simulink subsystem "GFDB"  (R2025b)
settings: Solver=VariableStepAuto  StartTime=0.0  StopTime=10.0  RelTol=1e-3
libraries: simulink x1
settings Model: Creator=diego  LastModifiedBy=ryanz
settings RTWCC: GPUComputeCapability=3.5

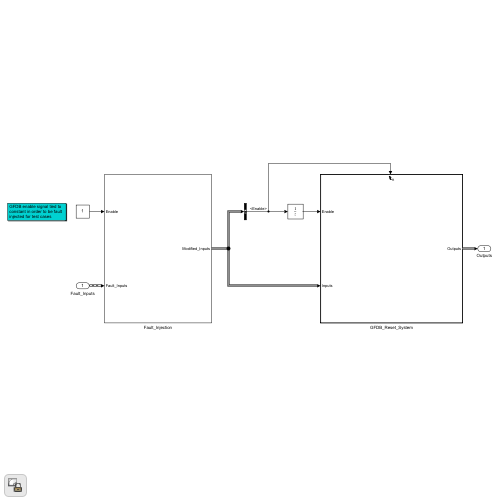
[thumbnail: Simulink's stored preview of the top-level diagram]
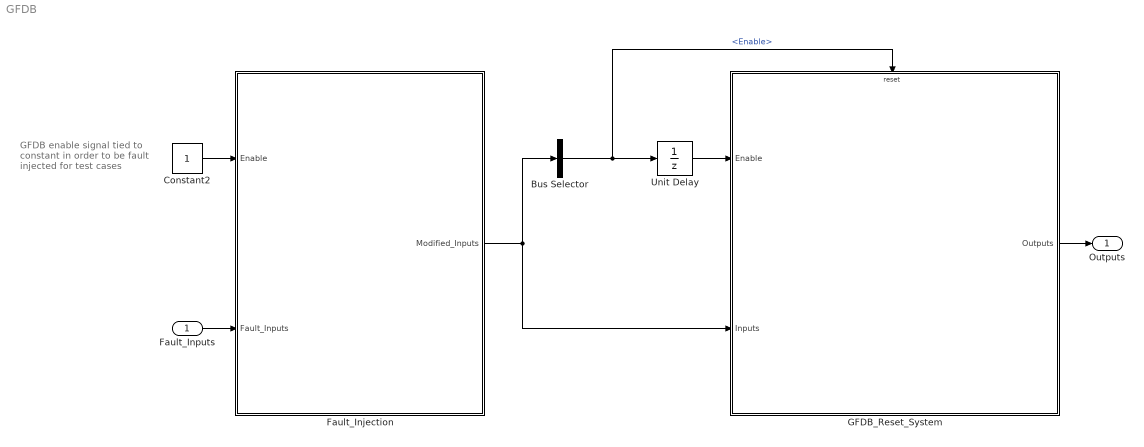
== system GFDB ==
  note: GFDB enable signal tied to constant in order to be fault injected for test cases
  Fault_Inputs : Inport
  Bus Selector : BusSelector  OutputSignals=Enable
  Constant2 : Constant
  Fault_Injection : Subsystem
  "GFDB_Reset_System " : Subsystem  TreatAsAtomicUnit=on
  Unit Delay : UnitDelay  SampleTime=-1  HasFrameUpgradeWarning=on
  Outputs : Outport
  wires:
  "GFDB_Reset_System "/1(Outputs) -> Outputs/1
  Fault_Inputs/1 -> Fault_Injection/2(Fault_Inputs)
  Constant2/1 -> Fault_Injection/1(Enable)
  Unit Delay/1 -> "GFDB_Reset_System "/1(Enable)
  Fault_Injection/1(Modified_Inputs) -> "GFDB_Reset_System "/2(Inputs), Bus Selector/1
  Bus Selector/1 -> "GFDB_Reset_System "/Reset, Unit Delay/1  "<Enable>"

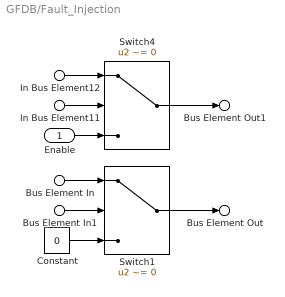
== system GFDB/Fault_Injection ==
  Enable : Inport
  Bus Element In1 : Inport  Port=2  PortName=Fault_Inputs  Element=Override_Isolation_State
  Bus Element In : Inport  Port=2  PortName=Fault_Inputs  Element=Fault_Value
  In Bus Element12 : Inport  Port=2  PortName=Fault_Inputs  Element=GFDB_EN
  In Bus Element11 : Inport  Port=2  PortName=Fault_Inputs  Element=Override_GFDB_EN
  Constant : Constant  Value=0
  Switch1 : Switch  Criteria=u2 ~= 0  SaturateOnIntegerOverflow=off  InputSameDT=off
  Switch4 : Switch  Criteria=u2 ~= 0  SaturateOnIntegerOverflow=off  InputSameDT=off
  Bus Element Out : Outport  PortName=Modified_Inputs  Element=Isolation_State
  Bus Element Out1 : Outport  PortName=Modified_Inputs  Element=Enable
  wires:
  Constant/1 -> Switch1/3
  Switch1/1 -> Bus Element Out/1
  Bus Element In/1 -> Switch1/1
  Bus Element In1/1 -> Switch1/2
  In Bus Element12/1 -> Switch4/1
  Switch4/1 -> Bus Element Out1/1
  In Bus Element11/1 -> Switch4/2
  Enable/1 -> Switch4/3

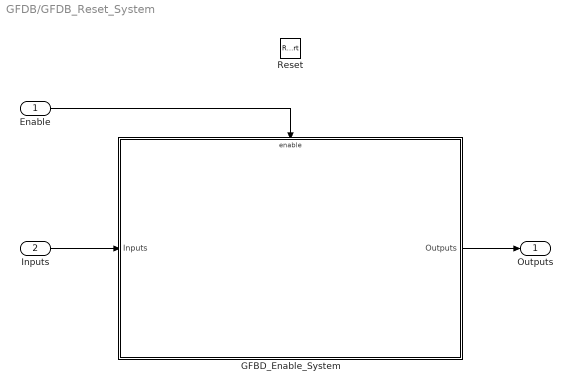
== system GFDB/GFDB_Reset_System  ==
  Enable : Inport
  Inputs : Inport  Port=2
  Reset : ResetPort  DisableCoverage=on  ResetTriggerType=falling
  "GFBD_Enable_System " : Subsystem  TreatAsAtomicUnit=on
  Outputs : Outport
  wires:
  Inputs/1 -> "GFBD_Enable_System "/1(Inputs)
  "GFBD_Enable_System "/1(Outputs) -> Outputs/1
  Enable/1 -> "GFBD_Enable_System "/Enable

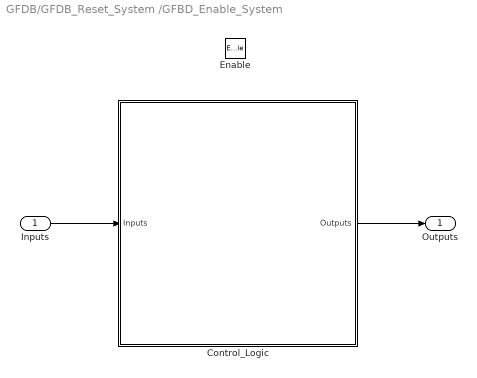
== system GFDB/GFDB_Reset_System /GFBD_Enable_System  ==
  Inputs : Inport
  Enable : EnablePort  StatesWhenEnabling=reset
  Control_Logic : Subsystem
  Outputs : Outport
  wires:
  Inputs/1 -> Control_Logic/1(Inputs)
  Control_Logic/1(Outputs) -> Outputs/1

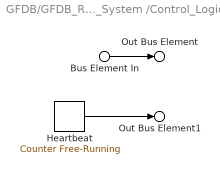
== system GFDB/GFDB_Reset_System /GFBD_Enable_System /Control_Logic ==
  Bus Element In : Inport  PortName=Inputs  Element=Isolation_State
  "Heartbeat " : simulink/Sources/Counter Free-Running  NumBits=32  tsamp=-1
  Out Bus Element : Outport  PortName=Outputs  Element=Isolation_State
  Out Bus Element1 : Outport  PortName=Outputs  Element=GFDB_Heartbeat
  wires:
  "Heartbeat "/1 -> Out Bus Element1/1
  Bus Element In/1 -> Out Bus Element/1
